simulink model "brain"  (Simulink 7.5)
settings: Solver=FixedStepDiscrete  StartTime=0.0  StopTime=inf  FixedStep=0.2  RelTol=1e-3
values from neighbouring files (symbols this model uses):
  Buoy1_Hue = 0.4    [brainconstants.m]    (also in brainconstants_David.m = 30)
  Buoy1_Saturation = 1.0    (= 1)    [brainconstants.m]    (also in brainconstants_David.m)
  Buoy1_Value = 0.45    [brainconstants.m]    (also in brainconstants_David.m)
  Buoy2_Hue = 0.0    (= 0)    [brainconstants.m]    (also in brainconstants_David.m = 80)
  Buoy2_Saturation = 1.0    (= 1)    [brainconstants.m]    (also in brainconstants_David.m)
  Buoy2_Value = 0.75    [brainconstants.m]    (also in brainconstants_David.m)
  Buoy_Max_Eccentricity = 0.7    [brainconstants.m]    (also in brainconstants_David.m = 1.2)
  Buoy_Max_Extent = 0.9    [brainconstants.m]    (also in brainconstants_David.m)
  Buoy_Min_Eccentricity = 0    [brainconstants.m]    (also in brainconstants_David.m)
  Buoy_Min_Extent = 0.7    [brainconstants.m]    (also in brainconstants_David.m = 0.1)
  Buoy_Strafe = 40    [brainconstants.m]    (also in brainconstants_David.m)
  Cam_Down_Strafe_XPos_Kd = 0.0    (= 0)    [brainconstants.m]    (also in brainconstants_David.m)
  Cam_Down_Strafe_XPos_Ki = 0.0    (= 0)    [brainconstants.m]    (also in brainconstants_David.m)
  Cam_Down_Strafe_XPos_Kp = -1.0    (= -1)    [brainconstants.m]    (also in brainconstants_David.m)
  Cam_Down_Yaw_XPos_Kd = 0.0    (= 0)    [brainconstants.m]    (also in brainconstants_David.m)
  Cam_Down_Yaw_XPos_Ki = 0.0    (= 0)    [brainconstants.m]    (also in brainconstants_David.m)
  Cam_Down_Yaw_XPos_Kp = 0.6    [brainconstants.m]    (also in brainconstants_David.m)
  Cam_Down_YPos_Kd = 0.0    (= 0)    [brainconstants.m]    (also in brainconstants_David.m)
  Cam_Down_YPos_Ki = 0.0    (= 0)    [brainconstants.m]    (also in brainconstants_David.m)
  Cam_Down_YPos_Kp = 0.75    [brainconstants.m]    (also in brainconstants_David.m)
  Cam_Forward_XPosition_Kd = 0.0    (= 0)    [brainconstants.m]    (also in brainconstants_David.m)
  Cam_Forward_XPosition_Ki = 0.0    (= 0)    [brainconstants.m]    (also in brainconstants_David.m)
  Cam_Forward_XPosition_Kp = 0.07    [brainconstants.m]    (also in brainconstants_David.m)
  Cam_Forward_YPosition_Kd = 0.0    (= 0)    [brainconstants.m]    (also in brainconstants_David.m)
  Cam_Forward_YPosition_Ki = 0.0    (= 0)    [brainconstants.m]    (also in brainconstants_David.m)
  Cam_Forward_YPosition_Kp = 0.8    [brainconstants.m]    (also in brainconstants_David.m)
  Depth_Kd = 0.0    (= 0)    [brainconstants.m]    (also in brainconstants_David.m)
  Depth_Ki = 0.0    (= 0)    [brainconstants.m]    (also in brainconstants_David.m)
  Depth_Kp = 75    [brainconstants.m]    (also in brainconstants_David.m)
  Heading_Forward_Velocity = 30    [brainconstants.m]    (also in brainconstants_David.m)
  Heading_Kd = 0.4    [brainconstants.m]    (also in brainconstants_David.m)
  Heading_Ki = 0.0    (= 0)    [brainconstants.m]    (also in brainconstants_David.m)
  Heading_Kp = 0.65    [brainconstants.m]    (also in brainconstants_David.m)
  Hedge_Hue = .4    (= 0.4)    [brainconstants.m]    (also in brainconstants_David.m)
  Hedge_Saturation = 1    [brainconstants.m]    (also in brainconstants_David.m)
  Hedge_Value = .75    (= 0.75)    [brainconstants.m]    (also in brainconstants_David.m)
  IMU_YawRate_Kd = 0.0    (= 0)    [brainconstants.m]    (also in brainconstants_David.m)
  IMU_YawRate_Ki = 0.0    (= 0)    [brainconstants.m]    (also in brainconstants_David.m)
  IMU_YawRate_Kp = 0.25    [brainconstants.m]    (also in brainconstants_David.m)
  IMU_YVel_Kd = 0.0    (= 0)    [brainconstants.m]    (also in brainconstants_David.m)
  IMU_YVel_Ki = 0.0    (= 0)    [brainconstants.m]    (also in brainconstants_David.m)
  IMU_YVel_Kp = 0.25    [brainconstants.m]    (also in brainconstants_David.m)
  Iter_Segment_Thresh = 60    [brainconstants.m]    (also in brainconstants_David.m)
  MissionPlan = [1 1 1 1 1 1 1 1 1 1 1 1 1 0 0 0 0 0 0 0]    [brainconstants.m]    (also in brainconstants_David.m)
  Track_Desired_Depth = 8    [brainconstants.m]    (also in brainconstants_David.m)
  Track_HueHigher = 0.75    [brainconstants.m]    (also in brainconstants_David.m)
  Track_HueLower = 0.4    [brainconstants.m]    (also in brainconstants_David.m)
  Track_Min_Eccentricity = 0.9    [brainconstants.m]    (also in brainconstants_David.m)
  Track_Saturation = 0.75    [brainconstants.m]    (also in brainconstants_David.m)
  Vision_Forward_Velocity = 15    [brainconstants.m]    (also in brainconstants_David.m)
undefined symbols (not defined in the file or in its folder): DiscIntNeverNeededParam, gray, Rec, SDTV, strel
libraries: vipconversions x32, simulink x26, vipgeotforms x9, vipstatistics x9, viptextngfix x7, vipmorphops x6, viptransforms x4, vipsnks x3, vipsrcs x1
(part 3 of 6)

== system brain/StateFlow Functions/StateFlowFunctions.GoStraight/PID Controller Relative Heading ==
  e : Inport
  Depth Discrete Derivative : simulink/Discrete/Discrete Derivative  SystemSampleTime=-1  gainval=1  ICPrevScaledInput=0.0  OutMin=[]  OutMax=[]  OutDataType=fixdt(1, 16)  OutScaling=2^-10  DoSatur=on
  Depth Discrete-Time Integrator : DiscreteIntegrator  gainval=1  SampleTime=-1  OutDataType=fixdt(1, 16)  OutScaling=2^0  LimitOutput=on  UpperSaturationLimit=10  LowerSaturationLimit=-10  ICPrevOutput=DiscIntNeverNeededParam  ICPrevScaledInput=DiscIntNeverNeededParam
  Sum : Sum  Inputs=+++  OutDataType=sfix(16)  OutScaling=2^0  SaturateOnIntegerOverflow=on  InputSameDT=on  OutDataTypeStr=Inherit: Same as first input
  Y-Accelerometer Derivative Gain : Gain  Gain=IMU_YVel_Kd  ParameterDataType=fixdt(1, 16)  ParameterScaling=2^0  OutDataType=fixdt(1, 16)  OutScaling=2^0
  Y-Accelerometer Integral Gain : Gain  Gain=IMU_YVel_Ki  ParameterDataType=fixdt(1, 16)  ParameterScaling=2^0  OutDataType=fixdt(1, 16)  OutScaling=2^0
  Y-Accelerometer Proportional Gain : Gain  Gain=IMU_YVel_Kp  ParameterDataType=fixdt(1, 16)  ParameterScaling=2^0  OutDataType=fixdt(1, 16)  OutScaling=2^0
  u : Outport
  wires:
  Y-Accelerometer Integral Gain/1 -> Depth Discrete-Time Integrator/1
  Y-Accelerometer Derivative Gain/1 -> Depth Discrete Derivative/1
  Depth Discrete Derivative/1 -> Sum/2
  Sum/1 -> u/1
  Y-Accelerometer Proportional Gain/1 -> Sum/1
  Depth Discrete-Time Integrator/1 -> Sum/3
  e/1 -> Y-Accelerometer Integral Gain/1, Y-Accelerometer Derivative Gain/1, Y-Accelerometer Proportional Gain/1

== system brain/StateFlow Functions/StateFlowFunctions.GoStraight/PID Controller YawRate ==
  e : Inport
  Heading Discrete Derivative : simulink/Discrete/Discrete Derivative  SystemSampleTime=-1  gainval=1  ICPrevScaledInput=0.0  OutMin=[]  OutMax=[]  OutDataType=fixdt(1, 16)  OutScaling=2^-10  DoSatur=off
  Heading Discrete-Time Integrator : DiscreteIntegrator  gainval=1  SampleTime=-1  OutDataType=fixdt(1, 16)  OutScaling=2^0  LimitOutput=on  UpperSaturationLimit=15  LowerSaturationLimit=-15  ICPrevOutput=DiscIntNeverNeededParam  ICPrevScaledInput=DiscIntNeverNeededParam
  Sum : Sum  Inputs=+++  OutDataType=sfix(16)  OutScaling=2^0  SaturateOnIntegerOverflow=on  InputSameDT=on  OutDataTypeStr=Inherit: Same as first input
  YawRate Derivative Gain : Gain  Gain=IMU_YawRate_Kd  ParameterDataType=fixdt(1, 16)  ParameterScaling=2^0  OutDataType=fixdt(1, 16)  OutScaling=2^0
  YawRate Integral Gain : Gain  Gain=IMU_YawRate_Ki  ParameterDataType=fixdt(1, 16)  ParameterScaling=2^0  OutDataType=fixdt(1, 16)  OutScaling=2^0
  YawRate Proportional Gain : Gain  Gain=IMU_YawRate_Kp  ParameterDataType=fixdt(1, 16)  ParameterScaling=2^0  OutDataType=fixdt(1, 16)  OutScaling=2^0
  u : Outport
  wires:
  YawRate Integral Gain/1 -> Heading Discrete-Time Integrator/1
  YawRate Derivative Gain/1 -> Heading Discrete Derivative/1
  Heading Discrete Derivative/1 -> Sum/2
  Sum/1 -> u/1
  YawRate Proportional Gain/1 -> Sum/1
  Heading Discrete-Time Integrator/1 -> Sum/3
  e/1 -> YawRate Integral Gain/1, YawRate Derivative Gain/1, YawRate Proportional Gain/1

== system brain/StateFlow Functions/StateFlowFunctions.JumpHedge.CameraForward_CenterOnBlobYaw/X-HeadingControl ==
  BuoyX : Inport  OutDataType=fixdt(1, 16)  OutScaling=2^0
  CenterX : Inport  Port=2  OutDataType=fixdt(1, 16)  OutScaling=2^0
  ForwardVel : Inport  Port=3
  Add : Sum  OutDataType=fixdt(1, 16)  OutScaling=2^-10
  Add1 : Sum  OutDataType=fixdt(1, 16)  OutScaling=2^-10
  Constant : Constant  Value=-1  OutDataType=fixdt(1, 16)  OutScaling=2^0  SampleTime=-1
  Data Type Conversion : DataTypeConversion  OutDataTypeMode=int8  OutDataType=fixdt(1, 16)  OutScaling=2^0  OutDataTypeStr=int8  SaturateOnIntegerOverflow=on
  Multiply : Product  Inputs=**  OutDataType=fixdt(1, 16)  OutScaling=2^-10
  PID Controller X Position : Subsystem  Description=PID
  Subtract : Sum  Inputs=+-  OutDataTypeMode=double  OutDataType=fixdt(1, 16)  OutScaling=2^-10  OutDataTypeStr=double
  ChangetoRight : Outport  OutDataType=fixdt(1, 16)  OutScaling=2^0
  ChangetoLeft : Outport  Port=2  OutDataType=fixdt(1, 16)  OutScaling=2^0
  wires:
  CenterX/1 -> Subtract/1
  BuoyX/1 -> Subtract/2
  Subtract/1 -> PID Controller X Position/1(e)  "Error"
  PID Controller X Position/1(u) -> Data Type Conversion/1
  Constant/1 -> Multiply/2
  Data Type Conversion/1 -> Multiply/1, Add/2
  Add/1 -> ChangetoRight/1
  Multiply/1 -> Add1/1
  ForwardVel/1 -> Add1/2, Add/1
  Add1/1 -> ChangetoLeft/1

== system brain/StateFlow Functions/StateFlowFunctions.JumpHedge.CameraForward_CenterOnBlobYaw/Y-DepthControl ==
  BuoyY : Inport  OutDataType=fixdt(1, 16)  OutScaling=2^0
  CenterY : Inport  Port=2  OutDataType=fixdt(1, 16)  OutScaling=2^0
  Data Type Conversion : DataTypeConversion  OutDataTypeMode=int8  OutDataType=fixdt(1, 16)  OutScaling=2^0  OutDataTypeStr=int8  SaturateOnIntegerOverflow=on
  PID Controller Y Position : Subsystem  Description=PID
  Subtract : Sum  Inputs=-+  OutDataTypeMode=double  OutDataType=fixdt(1, 16)  OutScaling=2^-10  OutDataTypeStr=double
  ChangetoVert : Outport  OutDataType=fixdt(1, 16)  OutScaling=2^0
  wires:
  CenterY/1 -> Subtract/1
  BuoyY/1 -> Subtract/2
  Subtract/1 -> PID Controller Y Position/1(e)  "Error"
  PID Controller Y Position/1(u) -> Data Type Conversion/1
  Data Type Conversion/1 -> ChangetoVert/1

== system brain/StateFlow Functions/StateFlowFunctions.JumpHedge.IndividualSegmentation/Threshold The Image ==
  LabelMatrix : Inport
  ref_colors : Inport  Port=2
  num_colors : Inport  Port=3
  H_Hue : Inport  Port=4
  H_Sat : Inport  Port=5
  H_Value : Inport  Port=6
  Choose Closest Color : Stateflow chart  TreatAsAtomicUnit=on
  Get Desired Color : Subsystem
  Relational Operator : RelationalOperator  Operator===  LogicOutDataTypeMode=boolean  LogicDataType=fixdt(0, 8)  OutDataTypeStr=boolean
  BW : Outport
  wires:
  Relational Operator/1 -> BW/1  "BW"
  ref_colors/1 -> Choose Closest Color/1(ref_colors)
  num_colors/1 -> Choose Closest Color/2(num_colors)
  Get Desired Color/1(L) -> Choose Closest Color/3(L)
  Get Desired Color/2(a) -> Choose Closest Color/4(a)
  Get Desired Color/3(b) -> Choose Closest Color/5(b)
  LabelMatrix/1 -> Relational Operator/1
  Choose Closest Color/1(index) -> Relational Operator/2
  H_Hue/1 -> Get Desired Color/1(B_Hue)
  H_Sat/1 -> Get Desired Color/2(B_Sat)
  H_Value/1 -> Get Desired Color/3(B_Value)

== system brain/StateFlow Functions/StateFlowFunctions.JumpHedge.IterativeSegmentation/Low Pass Filter ==
  R : Inport
  G : Inport  Port=2
  B : Inport  Port=3
  Low Pass Filter : Stateflow chart  TreatAsAtomicUnit=on
  Low Pass Filter1 : Stateflow chart  TreatAsAtomicUnit=on
  Low Pass Filter2 : Stateflow chart  TreatAsAtomicUnit=on
  R' : Outport
  G' : Outport  Port=2
  B' : Outport  Port=3
  wires:
  R/1 -> Low Pass Filter/1(I)
  G/1 -> Low Pass Filter1/1(I)
  B/1 -> Low Pass Filter2/1(I)
  Low Pass Filter1/1(Iout) -> G'/1
  Low Pass Filter2/1(Iout) -> B'/1
  Low Pass Filter/1(Iout) -> R'/1

== system brain/StateFlow Functions/StateFlowFunctions.JumpHedge.IterativeSegmentation/Segmentation ==
  L : Inport
  a : Inport  Port=2
  b : Inport  Port=3
  Dist_Thresh : Constant  Value=Iter_Segment_Thresh  OutDataType=fixdt(1, 16)  OutScaling=2^0  SampleTime=-1
  LabSegmentation : Stateflow chart  TreatAsAtomicUnit=on
  Reference Color Selection : Stateflow chart  TreatAsAtomicUnit=on
  Resize : Subsystem
  LabelMatrix : Outport
  num_colors : Outport  Port=2
  ref_colors : Outport  Port=3
  wires:
  L/1 -> Resize/1(In1), LabSegmentation/1(L)
  a/1 -> Resize/2(In2), LabSegmentation/2(a)
  b/1 -> Resize/3(In3), LabSegmentation/3(b)
  Resize/1(Out1) -> Reference Color Selection/1(L)
  Resize/2(Out2) -> Reference Color Selection/2(a)
  Resize/3(Out3) -> Reference Color Selection/3(b)
  Reference Color Selection/1(ref_colors) -> LabSegmentation/4(ref_colors), ref_colors/1
  Reference Color Selection/2(num_colors) -> LabSegmentation/5(num_colors), num_colors/1
  LabSegmentation/1(LabelMatrix) -> LabelMatrix/1
  Dist_Thresh/1 -> Reference Color Selection/4(Dist_Thresh)

== system brain/StateFlow Functions/StateFlowFunctions.MaintainDepth/PID Controller Depth S3 ==
  e : Inport
  Depth Derivative Gain : Gain  Gain=Depth_Kd  ParameterDataType=fixdt(1, 16)  ParameterScaling=2^0  OutDataType=fixdt(1, 16)  OutScaling=2^0
  Depth Discrete Derivative : simulink/Discrete/Discrete Derivative  SystemSampleTime=-1  gainval=1  ICPrevScaledInput=0.0  OutMin=[]  OutMax=[]  OutDataType=fixdt(1, 16)  OutScaling=2^-10  DoSatur=on
  Depth Discrete-Time Integrator : DiscreteIntegrator  gainval=1  SampleTime=-1  OutDataType=fixdt(1, 16)  OutScaling=2^0  LimitOutput=on  UpperSaturationLimit=10  LowerSaturationLimit=-10  ICPrevOutput=DiscIntNeverNeededParam  ICPrevScaledInput=DiscIntNeverNeededParam
  Depth Integral Gain : Gain  Gain=Depth_Ki  ParameterDataType=fixdt(1, 16)  ParameterScaling=2^0  OutDataType=fixdt(1, 16)  OutScaling=2^0
  Depth Proportional Gain : Gain  Gain=Depth_Kp  ParameterDataType=fixdt(1, 16)  ParameterScaling=2^0  OutDataType=fixdt(1, 16)  OutScaling=2^0
  Sum : Sum  Inputs=+++  OutDataType=sfix(16)  OutScaling=2^0  SaturateOnIntegerOverflow=on  InputSameDT=on  OutDataTypeStr=Inherit: Same as first input
  u : Outport
  wires:
  Depth Integral Gain/1 -> Depth Discrete-Time Integrator/1
  Depth Derivative Gain/1 -> Depth Discrete Derivative/1
  Depth Discrete Derivative/1 -> Sum/2
  Sum/1 -> u/1
  Depth Proportional Gain/1 -> Sum/1
  Depth Discrete-Time Integrator/1 -> Sum/3
  e/1 -> Depth Integral Gain/1, Depth Derivative Gain/1, Depth Proportional Gain/1

== system brain/StateFlow Functions/StateFlowFunctions.MaintainHeading/BigError S1 ==
  In1 : Inport  OutDataType=fixdt(1, 16)  OutScaling=2^0
  Action Port : ActionPort  PropagateVarSize=During execution  ActionType=then
  Add : Sum  Inputs=+-  OutDataType=fixdt(1, 16)  OutScaling=2^-10
  Constant : Constant  Value=360  OutDataType=fixdt(1, 16)  OutScaling=2^0  SampleTime=-1
  Constant1 : Constant  OutDataType=fixdt(1, 16)  OutScaling=2^0  SampleTime=-1
  Out1 : Outport  OutDataType=fixdt(1, 16)  OutScaling=2^0
  Out2 : Outport  Port=2  OutDataType=fixdt(1, 16)  OutScaling=2^0  OutputWhenDisabled=reset  InitialOutput=[0]
  wires:
  Constant1/1 -> Out2/1
  Add/1 -> Out1/1
  Constant/1 -> Add/2
  In1/1 -> Add/1

== system brain/StateFlow Functions/StateFlowFunctions.MaintainHeading/BigNegativeError S2 ==
  In1 : Inport  OutDataType=fixdt(1, 16)  OutScaling=2^0
  Action Port : ActionPort  PropagateVarSize=During execution  ActionType=elseif
  Add : Sum  OutDataType=fixdt(1, 16)  OutScaling=2^-10
  Constant : Constant  Value=360  OutDataType=fixdt(1, 16)  OutScaling=2^0  SampleTime=-1
  Constant1 : Constant  Value=2  OutDataType=fixdt(1, 16)  OutScaling=2^0  SampleTime=-1
  Out1 : Outport  OutDataType=fixdt(1, 16)  OutScaling=2^0
  Out2 : Outport  Port=2  OutDataType=fixdt(1, 16)  OutScaling=2^0  OutputWhenDisabled=reset  InitialOutput=[0]
  wires:
  Constant1/1 -> Out2/1
  Add/1 -> Out1/1
  Constant/1 -> Add/2
  In1/1 -> Add/1

== system brain/StateFlow Functions/StateFlowFunctions.MaintainHeading/PID Controller Heading S4 ==
  e : Inport
  Heading Derivative Gain : Gain  Gain=Heading_Kd  ParameterDataType=fixdt(1, 16)  ParameterScaling=2^0  OutDataType=fixdt(1, 16)  OutScaling=2^0
  Heading Discrete Derivative : simulink/Discrete/Discrete Derivative  SystemSampleTime=-1  gainval=1  ICPrevScaledInput=0.0  OutMin=[]  OutMax=[]  OutDataType=fixdt(1, 16)  OutScaling=2^-10  DoSatur=off
  Heading Discrete-Time Integrator : DiscreteIntegrator  gainval=1  SampleTime=-1  OutDataType=fixdt(1, 16)  OutScaling=2^0  LimitOutput=on  UpperSaturationLimit=15  LowerSaturationLimit=-15  ICPrevOutput=DiscIntNeverNeededParam  ICPrevScaledInput=DiscIntNeverNeededParam
  Heading Integral Gain : Gain  Gain=Heading_Ki  ParameterDataType=fixdt(1, 16)  ParameterScaling=2^0  OutDataType=fixdt(1, 16)  OutScaling=2^0
  Heading Proportional Gain : Gain  Gain=Heading_Kp  ParameterDataType=fixdt(1, 16)  ParameterScaling=2^0  OutDataType=fixdt(1, 16)  OutScaling=2^0
  Sum : Sum  Inputs=+++  OutDataType=sfix(16)  OutScaling=2^0  SaturateOnIntegerOverflow=on  InputSameDT=on  OutDataTypeStr=Inherit: Same as first input
  u : Outport
  wires:
  Heading Integral Gain/1 -> Heading Discrete-Time Integrator/1
  Heading Derivative Gain/1 -> Heading Discrete Derivative/1
  Heading Discrete Derivative/1 -> Sum/2
  Sum/1 -> u/1
  Heading Proportional Gain/1 -> Sum/1
  Heading Discrete-Time Integrator/1 -> Sum/3
  e/1 -> Heading Integral Gain/1, Heading Derivative Gain/1, Heading Proportional Gain/1

== system brain/StateFlow Functions/StateFlowFunctions.ValidationGate.LookforTrack/LookforTrack ==
  H : Inport
  S : Inport  Port=2  OutDataType=fixdt(1, 16)  OutScaling=2^0
  Blob Analysis : vipstatistics/Blob Analysis  Tag=vipblks_row_conv  DialogController=vipDDGCreate  DialogControllerArgs=DataTag35  area=off  centroid=off  bBox=off  majorAxis=off  minorAxis=off  angle=off  eccentricity=on  equivDiameterSq=off  extent=off  perimeter=off  maxBlobs=Max_Num_Blobs  warnIfNumBlobsExceeded=on  isCount=off  useMinArea=on  minArea=Min_Blob_Size  useMaxArea=on  maxArea=Max_Blob_Size  excludeBorderBlob=off  outDT=single  isOutVarDim=off  isFill=on  fillValues=-1  conn=8  isLabel=off  outputMode=Binary point scaling  outputWordLength=32  outputFracLength=16  firstCoeffMode=Binary point scaling  firstCoeffWordLength=16  firstCoeffFracLength=14  secondCoeffMode=Binary point scaling  secondCoeffWordLength=32  secondCoeffFracLength=16  accumMode=Binary point scaling  accumWordLength=32  accumFracLength=0  prodOutputMode=Binary point scaling  prodOutputWordLength=32  prodOutputFracLength=16  roundingMode=Floor  overflowMode=off
  CheckConditions : Stateflow chart  TreatAsAtomicUnit=on
  Constant : Constant  Value=Track_Min_Eccentricity  OutDataType=fixdt(1, 16)  OutScaling=2^0  SampleTime=-1
  Hue Higher Comparison : simulink/Logic and Bit Operations/Compare To Constant  SystemSampleTime=-1  relop=>  const=Track_HueHigher  LogicOutDataTypeMode=boolean  ZeroCross=off
  Hue Lower Comparison : simulink/Logic and Bit Operations/Compare To Constant  SystemSampleTime=-1  relop=<  const=Track_HueLower  LogicOutDataTypeMode=boolean  ZeroCross=off
  Logical Operator : Logic  Operator=OR  AllPortsSameDT=off  OutDataTypeMode=boolean  LogicDataType=fixdt(0, 8)  OutDataTypeStr=boolean
  Logical Operator1 : Logic  AllPortsSameDT=off  OutDataTypeMode=boolean  LogicDataType=fixdt(0, 8)  OutDataTypeStr=boolean
  Saturation Comparison : simulink/Logic and Bit Operations/Compare To Constant  SystemSampleTime=-1  relop=>  const=Track_Saturation  LogicOutDataTypeMode=boolean  ZeroCross=off
  BWout : Outport  OutDataType=fixdt(1, 16)  OutScaling=2^0
  Image : Outport  Port=2  OutDataType=fixdt(1, 16)  OutScaling=2^0
  wires:
  H/1 -> Hue Lower Comparison/1, Hue Higher Comparison/1
  Hue Lower Comparison/1 -> Logical Operator/1
  Hue Higher Comparison/1 -> Logical Operator/2
  Blob Analysis/1 -> CheckConditions/1(Eccent)
  S/1 -> Saturation Comparison/1
  Logical Operator/1 -> Logical Operator1/1
  Saturation Comparison/1 -> Logical Operator1/2
  Logical Operator1/1 -> Blob Analysis/1, BWout/1  "BW"
  Constant/1 -> CheckConditions/2(Track_Min_Eccentricity)
  CheckConditions/1(Image) -> Image/1

== system brain/StateFlow Functions/StateFlowFunctions.Buoys.ApproachBuoys.Buoy/Threshold The Image/Get Desired Color ==
  B_Hue : Inport  PortDimensions=1
  B_Sat : Inport  Port=2  PortDimensions=1
  B_Value : Inport  Port=3  PortDimensions=1
  Color Space  Conversion : vipconversions/Color Space  Conversion  conversion=Obsolete  conversionActive=HSV to R'G'B'  wp_str=D65  rec=Rec. 601 (SDTV)  sys=1125/60/2:1  imagePorts=Separate color signals
  Color Space  Conversion1 : vipconversions/Color Space  Conversion  conversion=Obsolete  conversionActive=sR'G'B' to L*a*b*  wp_str=D50  rec=Rec. 601 (SDTV)  sys=1125/60/2:1  imagePorts=Separate color signals
  L : Outport
  a : Outport  Port=2
  b : Outport  Port=3
  wires:
  B_Hue/1 -> Color Space  Conversion/1
  B_Sat/1 -> Color Space  Conversion/2
  B_Value/1 -> Color Space  Conversion/3
  Color Space  Conversion/1 -> Color Space  Conversion1/1
  Color Space  Conversion/2 -> Color Space  Conversion1/2
  Color Space  Conversion/3 -> Color Space  Conversion1/3
  Color Space  Conversion1/1 -> L/1
  Color Space  Conversion1/2 -> a/1
  Color Space  Conversion1/3 -> b/1

== system brain/StateFlow Functions/StateFlowFunctions.Buoys.ApproachBuoys.Buoy/X-HeadingControl/PID Controller X Position ==
  e : Inport
  Sum : Sum  Inputs=+++  OutDataType=sfix(16)  OutScaling=2^0  SaturateOnIntegerOverflow=on  InputSameDT=on  OutDataTypeStr=Inherit: Same as first input
  X-Buoy Derivative Gain : Gain  Gain=Cam_Forward_XPosition_Kd  ParameterDataType=fixdt(1, 16)  ParameterScaling=2^0  OutDataType=fixdt(1, 16)  OutScaling=2^0
  X-Buoy Discrete Derivative : simulink/Discrete/Discrete Derivative  SystemSampleTime=-1  gainval=1  ICPrevScaledInput=0.0  OutMin=[]  OutMax=[]  OutDataType=fixdt(1, 16)  OutScaling=2^-10  DoSatur=off
  X-Buoy Discrete-Time Integrator : DiscreteIntegrator  gainval=1  SampleTime=-1  OutDataType=fixdt(1, 16)  OutScaling=2^0  LimitOutput=on  UpperSaturationLimit=15  LowerSaturationLimit=-15  ICPrevOutput=DiscIntNeverNeededParam  ICPrevScaledInput=DiscIntNeverNeededParam
  X-Buoy Integral Gain : Gain  Gain=Cam_Forward_XPosition_Ki  ParameterDataType=fixdt(1, 16)  ParameterScaling=2^0  OutDataType=fixdt(1, 16)  OutScaling=2^0
  X-Buoy Proportional Gain : Gain  Gain=Cam_Forward_XPosition_Kp  ParameterDataType=fixdt(1, 16)  ParameterScaling=2^0  OutDataType=fixdt(1, 16)  OutScaling=2^0
  u : Outport
  wires:
  e/1 -> X-Buoy Proportional Gain/1, X-Buoy Derivative Gain/1, X-Buoy Integral Gain/1
  X-Buoy Discrete-Time Integrator/1 -> Sum/3
  X-Buoy Proportional Gain/1 -> Sum/1
  Sum/1 -> u/1
  X-Buoy Discrete Derivative/1 -> Sum/2
  X-Buoy Derivative Gain/1 -> X-Buoy Discrete Derivative/1
  X-Buoy Integral Gain/1 -> X-Buoy Discrete-Time Integrator/1

== system brain/StateFlow Functions/StateFlowFunctions.Buoys.ApproachBuoys.Buoy/Y-DepthControl/PID Controller Y Position ==
  e : Inport
  Sum : Sum  Inputs=+++  OutDataType=sfix(16)  OutScaling=2^0  SaturateOnIntegerOverflow=on  InputSameDT=on  OutDataTypeStr=Inherit: Same as first input
  Y-Buoy Derivative Gain : Gain  Gain=Cam_Forward_YPosition_Kd  ParameterDataType=fixdt(1, 16)  ParameterScaling=2^0  OutDataType=fixdt(1, 16)  OutScaling=2^0
  Y-Buoy Discrete Derivative : simulink/Discrete/Discrete Derivative  SystemSampleTime=-1  gainval=1  ICPrevScaledInput=0.0  OutMin=[]  OutMax=[]  OutDataType=fixdt(1, 16)  OutScaling=2^-10  DoSatur=off
  Y-Buoy Discrete-Time Integrator : DiscreteIntegrator  gainval=1  SampleTime=-1  OutDataType=fixdt(1, 16)  OutScaling=2^0  LimitOutput=on  UpperSaturationLimit=15  LowerSaturationLimit=-15  ICPrevOutput=DiscIntNeverNeededParam  ICPrevScaledInput=DiscIntNeverNeededParam
  Y-Buoy Integral Gain : Gain  Gain=Cam_Forward_YPosition_Ki  ParameterDataType=fixdt(1, 16)  ParameterScaling=2^0  OutDataType=fixdt(1, 16)  OutScaling=2^0
  Y-Buoy Proportional Gain : Gain  Gain=Cam_Forward_YPosition_Kp  ParameterDataType=fixdt(1, 16)  ParameterScaling=2^0  OutDataType=fixdt(1, 16)  OutScaling=2^0
  u : Outport
  wires:
  e/1 -> Y-Buoy Proportional Gain/1, Y-Buoy Derivative Gain/1, Y-Buoy Integral Gain/1
  Y-Buoy Discrete-Time Integrator/1 -> Sum/3
  Y-Buoy Proportional Gain/1 -> Sum/1
  Sum/1 -> u/1
  Y-Buoy Discrete Derivative/1 -> Sum/2
  Y-Buoy Derivative Gain/1 -> Y-Buoy Discrete Derivative/1
  Y-Buoy Integral Gain/1 -> Y-Buoy Discrete-Time Integrator/1

== system brain/StateFlow Functions/StateFlowFunctions.Buoys.ApproachBuoys.FindSecondBuoy.SecondBuoy/Threshold The Image/Get Desired Color ==
  B_Hue : Inport  PortDimensions=1
  B_Sat : Inport  Port=2  PortDimensions=1
  B_Value : Inport  Port=3  PortDimensions=1
  Color Space  Conversion : vipconversions/Color Space  Conversion  conversion=Obsolete  conversionActive=HSV to R'G'B'  wp_str=D65  rec=Rec. 601 (SDTV)  sys=1125/60/2:1  imagePorts=Separate color signals
  Color Space  Conversion1 : vipconversions/Color Space  Conversion  conversion=Obsolete  conversionActive=sR'G'B' to L*a*b*  wp_str=D50  rec=Rec. 601 (SDTV)  sys=1125/60/2:1  imagePorts=Separate color signals
  L : Outport
  a : Outport  Port=2
  b : Outport  Port=3
  wires:
  B_Hue/1 -> Color Space  Conversion/1
  B_Sat/1 -> Color Space  Conversion/2
  B_Value/1 -> Color Space  Conversion/3
  Color Space  Conversion/1 -> Color Space  Conversion1/1
  Color Space  Conversion/2 -> Color Space  Conversion1/2
  Color Space  Conversion/3 -> Color Space  Conversion1/3
  Color Space  Conversion1/1 -> L/1
  Color Space  Conversion1/2 -> a/1
  Color Space  Conversion1/3 -> b/1

== system brain/StateFlow Functions/StateFlowFunctions.Buoys.IterativeSegmentation/Segmentation/Resize ==
  In1 : Inport
  In2 : Inport  Port=2
  In3 : Inport  Port=3
  Resize : vipgeotforms/Resize  DialogController=vipDDGCreate  DialogControllerArgs=DataTag15  specify=Number of output rows and columns  rfactor=[]  outCols=25  outRows=25  outRowsCols=[60 80]  interp_method=Bilinear  antialias=on  useROI=off  roiFlag=off  prodOutputMode=Binary point scaling  prodOutputWordLength=32  prodOutputFracLength=10  roundingMode=Nearest  overflowMode=on
  Resize1 : vipgeotforms/Resize  DialogController=vipDDGCreate  DialogControllerArgs=DataTag16  specify=Number of output rows and columns  rfactor=[200 150]  outCols=25  outRows=25  outRowsCols=[60 80]  interp_method=Bilinear  antialias=on  useROI=off  roiFlag=off  prodOutputMode=Binary point scaling  prodOutputWordLength=32  prodOutputFracLength=10  roundingMode=Nearest  overflowMode=on
  Resize2 : vipgeotforms/Resize  DialogController=vipDDGCreate  DialogControllerArgs=DataTag17  specify=Number of output rows and columns  rfactor=[200 150]  outCols=25  outRows=25  outRowsCols=[60 80]  interp_method=Bilinear  antialias=on  useROI=off  roiFlag=off  prodOutputMode=Binary point scaling  prodOutputWordLength=32  prodOutputFracLength=10  roundingMode=Nearest  overflowMode=on
  Out1 : Outport
  Out2 : Outport  Port=2
  Out3 : Outport  Port=3
  wires:
  In1/1 -> Resize/1
  Resize/1 -> Out1/1
  In2/1 -> Resize1/1
  Resize1/1 -> Out2/1
  In3/1 -> Resize2/1
  Resize2/1 -> Out3/1

== system brain/StateFlow Functions/StateFlowFunctions.FollowOnePath.OnePath.CamDown_CenterOver_Yaw/X-Axis Control/PID Controller X Position ==
  e : Inport
  Sum : Sum  Inputs=+++  OutDataType=sfix(16)  OutScaling=2^0  SaturateOnIntegerOverflow=on  InputSameDT=on  OutDataTypeStr=Inherit: Same as first input
  X-Buoy Derivative Gain : Gain  Gain=Cam_Down_Yaw_XPos_Kd  ParameterDataType=fixdt(1, 16)  ParameterScaling=2^0  OutDataType=fixdt(1, 16)  OutScaling=2^0
  X-Buoy Discrete Derivative : simulink/Discrete/Discrete Derivative  SystemSampleTime=-1  gainval=1  ICPrevScaledInput=0.0  OutMin=[]  OutMax=[]  OutDataType=fixdt(1, 16)  OutScaling=2^-10  DoSatur=off
  X-Buoy Discrete-Time Integrator : DiscreteIntegrator  gainval=1  SampleTime=-1  OutDataType=fixdt(1, 16)  OutScaling=2^0  LimitOutput=on  UpperSaturationLimit=15  LowerSaturationLimit=-15  ICPrevOutput=DiscIntNeverNeededParam  ICPrevScaledInput=DiscIntNeverNeededParam
  X-Buoy Integral Gain : Gain  Gain=Cam_Down_Yaw_XPos_Ki  ParameterDataType=fixdt(1, 16)  ParameterScaling=2^0  OutDataType=fixdt(1, 16)  OutScaling=2^0
  X-Buoy Proportional Gain : Gain  Gain=Cam_Down_Yaw_XPos_Kp  ParameterDataType=fixdt(1, 16)  ParameterScaling=2^0  OutDataType=fixdt(1, 16)  OutScaling=2^0
  u : Outport
  wires:
  e/1 -> X-Buoy Proportional Gain/1, X-Buoy Derivative Gain/1, X-Buoy Integral Gain/1
  X-Buoy Discrete-Time Integrator/1 -> Sum/3
  X-Buoy Proportional Gain/1 -> Sum/1
  Sum/1 -> u/1
  X-Buoy Discrete Derivative/1 -> Sum/2
  X-Buoy Derivative Gain/1 -> X-Buoy Discrete Derivative/1
  X-Buoy Integral Gain/1 -> X-Buoy Discrete-Time Integrator/1

== system brain/StateFlow Functions/StateFlowFunctions.FollowOnePath.OnePath.CamDown_CenterOver_Yaw/Y-Axis Control/PID Controller Y Axis ==
  e : Inport
  Sum : Sum  Inputs=+++  OutDataType=sfix(16)  OutScaling=2^0  SaturateOnIntegerOverflow=on  InputSameDT=on  OutDataTypeStr=Inherit: Same as first input
  Y-Blob Derivative Gain : Gain  Gain=Cam_Down_YPos_Kd  ParameterDataType=fixdt(1, 16)  ParameterScaling=2^0  OutDataType=fixdt(1, 16)  OutScaling=2^0
  Y-Blob Integral Gain : Gain  Gain=Cam_Down_YPos_Ki  ParameterDataType=fixdt(1, 16)  ParameterScaling=2^0  OutDataType=fixdt(1, 16)  OutScaling=2^0
  Y-Blob Proportional Gain : Gain  Gain=Cam_Down_YPos_Kp  ParameterDataType=fixdt(1, 16)  ParameterScaling=2^0  OutDataType=fixdt(1, 16)  OutScaling=2^0
  Y-Buoy Discrete Derivative : simulink/Discrete/Discrete Derivative  SystemSampleTime=-1  gainval=1  ICPrevScaledInput=0.0  OutMin=[]  OutMax=[]  OutDataType=fixdt(1, 16)  OutScaling=2^-10  DoSatur=off
  Y-Buoy Discrete-Time Integrator : DiscreteIntegrator  gainval=1  SampleTime=-1  OutDataType=fixdt(1, 16)  OutScaling=2^0  LimitOutput=on  UpperSaturationLimit=15  LowerSaturationLimit=-15  ICPrevOutput=DiscIntNeverNeededParam  ICPrevScaledInput=DiscIntNeverNeededParam
  u : Outport
  wires:
  e/1 -> Y-Blob Proportional Gain/1, Y-Blob Derivative Gain/1, Y-Blob Integral Gain/1
  Y-Buoy Discrete-Time Integrator/1 -> Sum/3
  Y-Blob Proportional Gain/1 -> Sum/1
  Sum/1 -> u/1
  Y-Buoy Discrete Derivative/1 -> Sum/2
  Y-Blob Derivative Gain/1 -> Y-Buoy Discrete Derivative/1
  Y-Blob Integral Gain/1 -> Y-Buoy Discrete-Time Integrator/1

== system brain/StateFlow Functions/StateFlowFunctions.FollowOnePath.OnePath.CenterOver_Strafe/X-Axis Control/PID Controller X Position ==
  e : Inport
  CamDown Strafe XPos Derivative Gain : Gain  Gain=Cam_Down_Strafe_XPos_Kd  ParameterDataType=fixdt(1, 16)  ParameterScaling=2^0  OutDataType=fixdt(1, 16)  OutScaling=2^0
  CamDown Strafe XPos Integral Gain : Gain  Gain=Cam_Down_Strafe_XPos_Ki  ParameterDataType=fixdt(1, 16)  ParameterScaling=2^0  OutDataType=fixdt(1, 16)  OutScaling=2^0
  CamDown Strafe XPos Proportional Gain : Gain  Gain=Cam_Down_Strafe_XPos_Kp  ParameterDataType=fixdt(1, 16)  ParameterScaling=2^0  OutDataType=fixdt(1, 16)  OutScaling=2^0
  Sum : Sum  Inputs=+++  OutDataType=sfix(16)  OutScaling=2^0  SaturateOnIntegerOverflow=on  InputSameDT=on  OutDataTypeStr=Inherit: Same as first input
  X-Buoy Discrete Derivative : simulink/Discrete/Discrete Derivative  SystemSampleTime=-1  gainval=1  ICPrevScaledInput=0.0  OutMin=[]  OutMax=[]  OutDataType=fixdt(1, 16)  OutScaling=2^-10  DoSatur=off
  X-Buoy Discrete-Time Integrator : DiscreteIntegrator  gainval=1  SampleTime=-1  OutDataType=fixdt(1, 16)  OutScaling=2^0  LimitOutput=on  UpperSaturationLimit=15  LowerSaturationLimit=-15  ICPrevOutput=DiscIntNeverNeededParam  ICPrevScaledInput=DiscIntNeverNeededParam
  u : Outport
  wires:
  e/1 -> CamDown Strafe XPos Proportional Gain/1, CamDown Strafe XPos Derivative Gain/1, CamDown Strafe XPos Integral Gain/1
  X-Buoy Discrete-Time Integrator/1 -> Sum/3
  CamDown Strafe XPos Proportional Gain/1 -> Sum/1
  Sum/1 -> u/1
  X-Buoy Discrete Derivative/1 -> Sum/2
  CamDown Strafe XPos Derivative Gain/1 -> X-Buoy Discrete Derivative/1
  CamDown Strafe XPos Integral Gain/1 -> X-Buoy Discrete-Time Integrator/1

== system brain/StateFlow Functions/StateFlowFunctions.FollowOnePath.OnePath.CenterOver_Strafe/Y-Axis Control/PID Controller Y Axis ==
  e : Inport
  Sum : Sum  Inputs=+++  OutDataType=sfix(16)  OutScaling=2^0  SaturateOnIntegerOverflow=on  InputSameDT=on  OutDataTypeStr=Inherit: Same as first input
  Y-Buoy Derivative Gain : Gain  Gain=Cam_Down_YPos_Kd  ParameterDataType=fixdt(1, 16)  ParameterScaling=2^0  OutDataType=fixdt(1, 16)  OutScaling=2^0
  Y-Buoy Discrete Derivative : simulink/Discrete/Discrete Derivative  SystemSampleTime=-1  gainval=1  ICPrevScaledInput=0.0  OutMin=[]  OutMax=[]  OutDataType=fixdt(1, 16)  OutScaling=2^-10  DoSatur=off
  Y-Buoy Discrete-Time Integrator : DiscreteIntegrator  gainval=1  SampleTime=-1  OutDataType=fixdt(1, 16)  OutScaling=2^0  LimitOutput=on  UpperSaturationLimit=15  LowerSaturationLimit=-15  ICPrevOutput=DiscIntNeverNeededParam  ICPrevScaledInput=DiscIntNeverNeededParam
  Y-Buoy Integral Gain : Gain  Gain=Cam_Down_YPos_Ki  ParameterDataType=fixdt(1, 16)  ParameterScaling=2^0  OutDataType=fixdt(1, 16)  OutScaling=2^0
  Y-Buoy Proportional Gain : Gain  Gain=Cam_Down_YPos_Kp  ParameterDataType=fixdt(1, 16)  ParameterScaling=2^0  OutDataType=fixdt(1, 16)  OutScaling=2^0
  u : Outport
  wires:
  e/1 -> Y-Buoy Proportional Gain/1, Y-Buoy Derivative Gain/1, Y-Buoy Integral Gain/1
  Y-Buoy Discrete-Time Integrator/1 -> Sum/3
  Y-Buoy Proportional Gain/1 -> Sum/1
  Sum/1 -> u/1
  Y-Buoy Discrete Derivative/1 -> Sum/2
  Y-Buoy Derivative Gain/1 -> Y-Buoy Discrete Derivative/1
  Y-Buoy Integral Gain/1 -> Y-Buoy Discrete-Time Integrator/1

== system brain/StateFlow Functions/StateFlowFunctions.JumpHedge.CameraForward_CenterOnBlobYaw/X-HeadingControl/PID Controller X Position ==
  e : Inport
  Sum : Sum  Inputs=+++  OutDataType=sfix(16)  OutScaling=2^0  SaturateOnIntegerOverflow=on  InputSameDT=on  OutDataTypeStr=Inherit: Same as first input
  X-Buoy Derivative Gain : Gain  Gain=Cam_Forward_XPosition_Kd  ParameterDataType=fixdt(1, 16)  ParameterScaling=2^0  OutDataType=fixdt(1, 16)  OutScaling=2^0
  X-Buoy Discrete Derivative : simulink/Discrete/Discrete Derivative  SystemSampleTime=-1  gainval=1  ICPrevScaledInput=0.0  OutMin=[]  OutMax=[]  OutDataType=fixdt(1, 16)  OutScaling=2^-10  DoSatur=off
  X-Buoy Discrete-Time Integrator : DiscreteIntegrator  gainval=1  SampleTime=-1  OutDataType=fixdt(1, 16)  OutScaling=2^0  LimitOutput=on  UpperSaturationLimit=15  LowerSaturationLimit=-15  ICPrevOutput=DiscIntNeverNeededParam  ICPrevScaledInput=DiscIntNeverNeededParam
  X-Buoy Integral Gain : Gain  Gain=Cam_Forward_XPosition_Ki  ParameterDataType=fixdt(1, 16)  ParameterScaling=2^0  OutDataType=fixdt(1, 16)  OutScaling=2^0
  X-Buoy Proportional Gain : Gain  Gain=Cam_Forward_XPosition_Kp  ParameterDataType=fixdt(1, 16)  ParameterScaling=2^0  OutDataType=fixdt(1, 16)  OutScaling=2^0
  u : Outport
  wires:
  e/1 -> X-Buoy Proportional Gain/1, X-Buoy Derivative Gain/1, X-Buoy Integral Gain/1
  X-Buoy Discrete-Time Integrator/1 -> Sum/3
  X-Buoy Proportional Gain/1 -> Sum/1
  Sum/1 -> u/1
  X-Buoy Discrete Derivative/1 -> Sum/2
  X-Buoy Derivative Gain/1 -> X-Buoy Discrete Derivative/1
  X-Buoy Integral Gain/1 -> X-Buoy Discrete-Time Integrator/1

== system brain/StateFlow Functions/StateFlowFunctions.JumpHedge.CameraForward_CenterOnBlobYaw/Y-DepthControl/PID Controller Y Position ==
  e : Inport
  Sum : Sum  Inputs=+++  OutDataType=sfix(16)  OutScaling=2^0  SaturateOnIntegerOverflow=on  InputSameDT=on  OutDataTypeStr=Inherit: Same as first input
  Y-Buoy Derivative Gain : Gain  Gain=Cam_Forward_YPosition_Kd  ParameterDataType=fixdt(1, 16)  ParameterScaling=2^0  OutDataType=fixdt(1, 16)  OutScaling=2^0
  Y-Buoy Discrete Derivative : simulink/Discrete/Discrete Derivative  SystemSampleTime=-1  gainval=1  ICPrevScaledInput=0.0  OutMin=[]  OutMax=[]  OutDataType=fixdt(1, 16)  OutScaling=2^-10  DoSatur=off
  Y-Buoy Discrete-Time Integrator : DiscreteIntegrator  gainval=1  SampleTime=-1  OutDataType=fixdt(1, 16)  OutScaling=2^0  LimitOutput=on  UpperSaturationLimit=15  LowerSaturationLimit=-15  ICPrevOutput=DiscIntNeverNeededParam  ICPrevScaledInput=DiscIntNeverNeededParam
  Y-Buoy Integral Gain : Gain  Gain=Cam_Forward_YPosition_Ki  ParameterDataType=fixdt(1, 16)  ParameterScaling=2^0  OutDataType=fixdt(1, 16)  OutScaling=2^0
  Y-Buoy Proportional Gain : Gain  Gain=Cam_Forward_YPosition_Kp  ParameterDataType=fixdt(1, 16)  ParameterScaling=2^0  OutDataType=fixdt(1, 16)  OutScaling=2^0
  u : Outport
  wires:
  e/1 -> Y-Buoy Proportional Gain/1, Y-Buoy Derivative Gain/1, Y-Buoy Integral Gain/1
  Y-Buoy Discrete-Time Integrator/1 -> Sum/3
  Y-Buoy Proportional Gain/1 -> Sum/1
  Sum/1 -> u/1
  Y-Buoy Discrete Derivative/1 -> Sum/2
  Y-Buoy Derivative Gain/1 -> Y-Buoy Discrete Derivative/1
  Y-Buoy Integral Gain/1 -> Y-Buoy Discrete-Time Integrator/1

== system brain/StateFlow Functions/StateFlowFunctions.JumpHedge.IndividualSegmentation/Threshold The Image/Get Desired Color ==
  B_Hue : Inport  PortDimensions=1
  B_Sat : Inport  Port=2  PortDimensions=1
  B_Value : Inport  Port=3  PortDimensions=1
  Color Space  Conversion : vipconversions/Color Space  Conversion  conversion=Obsolete  conversionActive=HSV to R'G'B'  wp_str=D65  rec=Rec. 601 (SDTV)  sys=1125/60/2:1  imagePorts=Separate color signals
  Color Space  Conversion1 : vipconversions/Color Space  Conversion  conversion=Obsolete  conversionActive=sR'G'B' to L*a*b*  wp_str=D50  rec=Rec. 601 (SDTV)  sys=1125/60/2:1  imagePorts=Separate color signals
  L : Outport
  a : Outport  Port=2
  b : Outport  Port=3
  wires:
  B_Hue/1 -> Color Space  Conversion/1
  B_Sat/1 -> Color Space  Conversion/2
  B_Value/1 -> Color Space  Conversion/3
  Color Space  Conversion/1 -> Color Space  Conversion1/1
  Color Space  Conversion/2 -> Color Space  Conversion1/2
  Color Space  Conversion/3 -> Color Space  Conversion1/3
  Color Space  Conversion1/1 -> L/1
  Color Space  Conversion1/2 -> a/1
  Color Space  Conversion1/3 -> b/1

== system brain/StateFlow Functions/StateFlowFunctions.JumpHedge.IterativeSegmentation/Segmentation/Resize ==
  In1 : Inport
  In2 : Inport  Port=2
  In3 : Inport  Port=3
  Resize : vipgeotforms/Resize  DialogController=vipDDGCreate  DialogControllerArgs=DataTag29  specify=Number of output rows and columns  rfactor=[]  outCols=25  outRows=25  outRowsCols=[60 80]  interp_method=Bilinear  antialias=on  useROI=off  roiFlag=off  prodOutputMode=Binary point scaling  prodOutputWordLength=32  prodOutputFracLength=10  roundingMode=Nearest  overflowMode=on
  Resize1 : vipgeotforms/Resize  DialogController=vipDDGCreate  DialogControllerArgs=DataTag30  specify=Number of output rows and columns  rfactor=[200 150]  outCols=25  outRows=25  outRowsCols=[60 80]  interp_method=Bilinear  antialias=on  useROI=off  roiFlag=off  prodOutputMode=Binary point scaling  prodOutputWordLength=32  prodOutputFracLength=10  roundingMode=Nearest  overflowMode=on
  Resize2 : vipgeotforms/Resize  DialogController=vipDDGCreate  DialogControllerArgs=DataTag31  specify=Number of output rows and columns  rfactor=[200 150]  outCols=25  outRows=25  outRowsCols=[60 80]  interp_method=Bilinear  antialias=on  useROI=off  roiFlag=off  prodOutputMode=Binary point scaling  prodOutputWordLength=32  prodOutputFracLength=10  roundingMode=Nearest  overflowMode=on
  Out1 : Outport
  Out2 : Outport  Port=2
  Out3 : Outport  Port=3
  wires:
  In1/1 -> Resize/1
  Resize/1 -> Out1/1
  In2/1 -> Resize1/1
  Resize1/1 -> Out2/1
  In3/1 -> Resize2/1
  Resize2/1 -> Out3/1
